simulink library "STATE_BIO_MASTER"  (Simulink 8.6)
settings: Solver=ode45  StartTime=0.0  StopTime=10.0  RelTol=1e-3
libraries: cdsBitwise x48, cdsEpicsIn x41, cdsFunctionCall x10, cdsEpicsOut x7
(part 1 of 2)
settings Model: Creator=controls  LastModifiedBy=controls

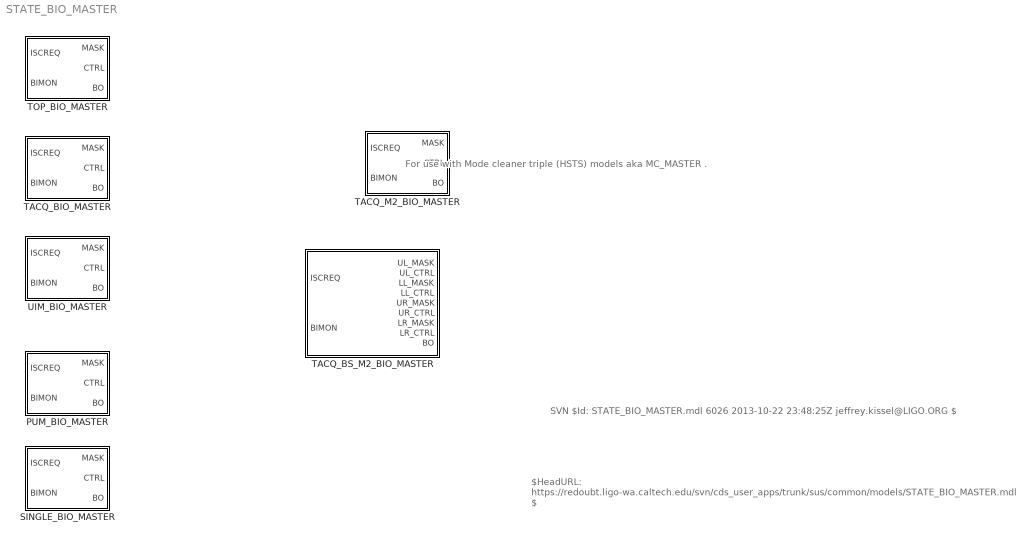
== system STATE_BIO_MASTER ==
  note: $HeadURL: https://redoubt.ligo-wa.caltech.edu/svn/cds_user_apps/trunk/sus/common/models/STATE_BIO_MASTER.mdl $
  note: For use with Mode cleaner triple (HSTS) models aka MC_MASTER
      |
      |
      |
      |
      |
      |
      |
      |
      |
      | .
  note: SVN $Id: STATE_BIO_MASTER.mdl 6026 2013-10-22 23:48:25Z jeffrey.kissel@LIGO.ORG $
  PUM_BIO_MASTER : Subsystem
  SINGLE_BIO_MASTER : Subsystem
  TACQ_BIO_MASTER : Subsystem
  TACQ_BS_M2_BIO_MASTER : Subsystem
  TACQ_M2_BIO_MASTER : Subsystem
  TOP_BIO_MASTER : Subsystem
  UIM_BIO_MASTER : Subsystem

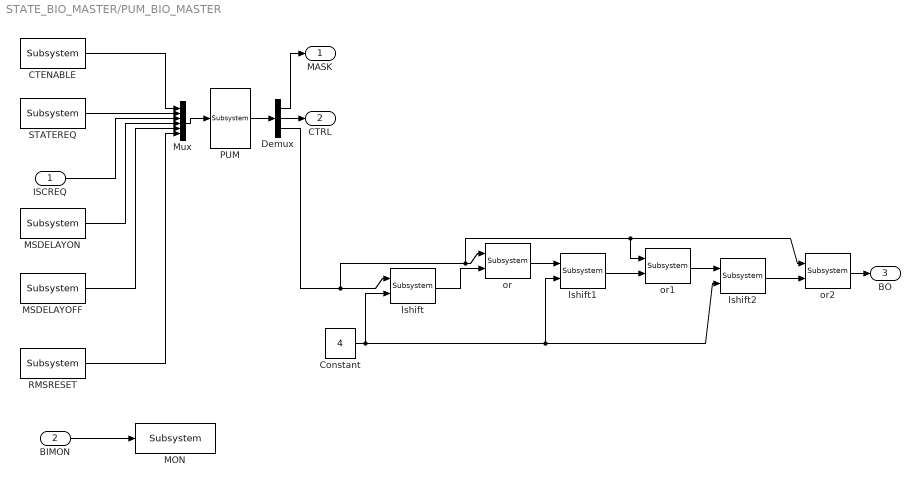
== system STATE_BIO_MASTER/PUM_BIO_MASTER ==
  ISCREQ : Inport
  BIMON : Inport  Port=2
  CTENABLE : cdsEpicsIn/Subsystem  Tag=cdsEpicsIn  Description=|
      | Purpose:                                                                              
      | Create an EPICS input channel connection to the FE realtime controls.                 
      |                                                                                       
      | Operation:                                                                            
      | Outputs value from an EPICS ai record. Value is floating point with a precision of 3..
      |                                                                                       
      | Usage:                                                                                
      | Name the part with the desired EPICS channel name.
      settings: AttributesFormatString=%<Tag>
  Constant : Constant  Value=4
  Demux : Demux  Outputs=3
  MON : cdsEpicsOut/Subsystem  Tag=cdsEpicsOutput  Description=|
      | Purpose:                                          
      | Output a FE signal to an EPICS channel.           
      |                                                   
      | Operation:                                        
      | Takes input value and passes it to EPICS record.  
      |                                                   
      | Usage:                                            
      | Name the part with the desired EPICS rrecord name.
      settings: AttributesFormatString=%<Tag>
  MSDELAYOFF : cdsEpicsIn/Subsystem  Tag=cdsEpicsIn  Description=|
      | Purpose:                                                                              
      | Create an EPICS input channel connection to the FE realtime controls.                 
      |                                                                                       
      | Operation:                                                                            
      | Outputs value from an EPICS ai record. Value is floating point with a precision of 3..
      |                                                                                       
      | Usage:                                                                                
      | Name the part with the desired EPICS channel name.
      settings: AttributesFormatString=%<Tag>
  MSDELAYON : cdsEpicsIn/Subsystem  Tag=cdsEpicsIn  Description=|
      | Purpose:                                                                              
      | Create an EPICS input channel connection to the FE realtime controls.                 
      |                                                                                       
      | Operation:                                                                            
      | Outputs value from an EPICS ai record. Value is floating point with a precision of 3..
      |                                                                                       
      | Usage:                                                                                
      | Name the part with the desired EPICS channel name.
      settings: AttributesFormatString=%<Tag>
  Mux : Mux  Inputs=6
  PUM : cdsFunctionCall/Subsystem  Tag=cdsFunctionCall  Description=inline PUM $SUS_SRC/CD_STATE_MACHINE.c
      settings: AttributesFormatString=%<Tag>
  RMSRESET : cdsEpicsIn/Subsystem  Tag=cdsEpicsIn  Description=|
      | Purpose:                                                                              
      | Create an EPICS input channel connection to the FE realtime controls.                 
      |                                                                                       
      | Operation:                                                                            
      | Outputs value from an EPICS ai record. Value is floating point with a precision of 3..
      |                                                                                       
      | Usage:                                                                                
      | Name the part with the desired EPICS channel name.
      settings: AttributesFormatString=%<Tag>
  STATEREQ : cdsEpicsIn/Subsystem  Tag=cdsEpicsIn  Description=|
      | Purpose:                                                                              
      | Create an EPICS input channel connection to the FE realtime controls.                 
      |                                                                                       
      | Operation:                                                                            
      | Outputs value from an EPICS ai record. Value is floating point with a precision of 3..
      |                                                                                       
      | Usage:                                                                                
      | Name the part with the desired EPICS channel name.
      settings: AttributesFormatString=%<Tag>
  lshift : cdsBitwise/Subsystem  Tag=cdsBitwise
      settings: AttributesFormatString=%<Tag>
  lshift1 : cdsBitwise/Subsystem  Tag=cdsBitwise
      settings: AttributesFormatString=%<Tag>
  lshift2 : cdsBitwise/Subsystem  Tag=cdsBitwise
      settings: AttributesFormatString=%<Tag>
  or : cdsBitwise/Subsystem  Tag=cdsBitwise
      settings: AttributesFormatString=%<Tag>
  or1 : cdsBitwise/Subsystem  Tag=cdsBitwise
      settings: AttributesFormatString=%<Tag>
  or2 : cdsBitwise/Subsystem  Tag=cdsBitwise
      settings: AttributesFormatString=%<Tag>
  MASK : Outport
  CTRL : Outport  Port=2
  BO : Outport  Port=3
  wires:
  PUM/1 -> Demux/1
  Mux/1 -> PUM/1
  CTENABLE/1 -> Mux/1
  STATEREQ/1 -> Mux/2
  ISCREQ/1 -> Mux/3
  MSDELAYON/1 -> Mux/4
  Demux/1 -> MASK/1
  Demux/2 -> CTRL/1
  BIMON/1 -> MON/1
  RMSRESET/1 -> Mux/6
  MSDELAYOFF/1 -> Mux/5
  Constant/1 -> lshift/2, lshift1/2, lshift2/2
  lshift/1 -> or/2
  or/1 -> lshift1/1
  lshift1/1 -> or1/2
  or1/1 -> lshift2/1
  lshift2/1 -> or2/2
  Demux/3 -> lshift/1, or/1, or1/1, or2/1
  or2/1 -> BO/1

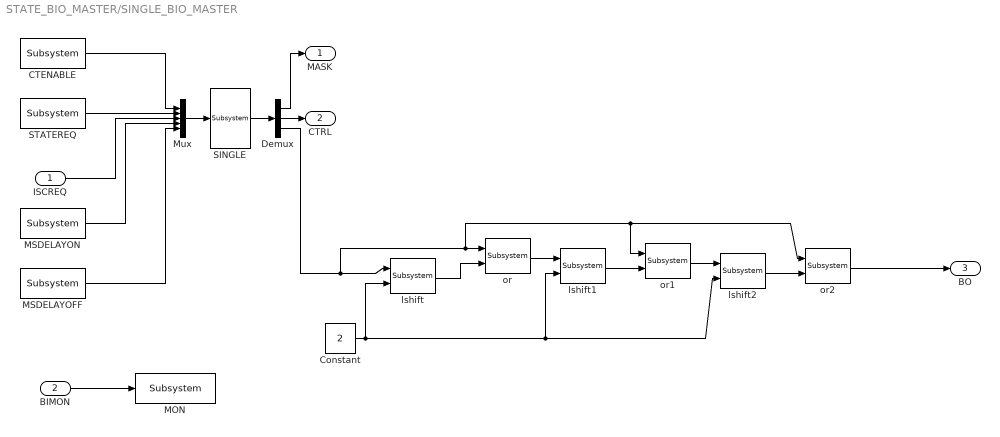
== system STATE_BIO_MASTER/SINGLE_BIO_MASTER ==
  ISCREQ : Inport
  BIMON : Inport  Port=2
  CTENABLE : cdsEpicsIn/Subsystem  Tag=cdsEpicsIn  Description=|
      | Purpose:                                                                              
      | Create an EPICS input channel connection to the FE realtime controls.                 
      |                                                                                       
      | Operation:                                                                            
      | Outputs value from an EPICS ai record. Value is floating point with a precision of 3..
      |                                                                                       
      | Usage:                                                                                
      | Name the part with the desired EPICS channel name.
      settings: AttributesFormatString=%<Tag>
  Constant : Constant  Value=2
  Demux : Demux  Outputs=3
  MON : cdsEpicsOut/Subsystem  Tag=cdsEpicsOutput  Description=|
      | Purpose:                                          
      | Output a FE signal to an EPICS channel.           
      |                                                   
      | Operation:                                        
      | Takes input value and passes it to EPICS record.  
      |                                                   
      | Usage:                                            
      | Name the part with the desired EPICS rrecord name.
      settings: AttributesFormatString=%<Tag>
  MSDELAYOFF : cdsEpicsIn/Subsystem  Tag=cdsEpicsIn  Description=|
      | Purpose:                                                                              
      | Create an EPICS input channel connection to the FE realtime controls.                 
      |                                                                                       
      | Operation:                                                                            
      | Outputs value from an EPICS ai record. Value is floating point with a precision of 3..
      |                                                                                       
      | Usage:                                                                                
      | Name the part with the desired EPICS channel name.
      settings: AttributesFormatString=%<Tag>
  MSDELAYON : cdsEpicsIn/Subsystem  Tag=cdsEpicsIn  Description=|
      | Purpose:                                                                              
      | Create an EPICS input channel connection to the FE realtime controls.                 
      |                                                                                       
      | Operation:                                                                            
      | Outputs value from an EPICS ai record. Value is floating point with a precision of 3..
      |                                                                                       
      | Usage:                                                                                
      | Name the part with the desired EPICS channel name.
      settings: AttributesFormatString=%<Tag>
  Mux : Mux  Inputs=5
  SINGLE : cdsFunctionCall/Subsystem  Tag=cdsFunctionCall  Description=inline SINGLE $SUS_SRC/CD_STATE_MACHINE.c
      settings: AttributesFormatString=%<Tag>
  STATEREQ : cdsEpicsIn/Subsystem  Tag=cdsEpicsIn  Description=|
      | Purpose:                                                                              
      | Create an EPICS input channel connection to the FE realtime controls.                 
      |                                                                                       
      | Operation:                                                                            
      | Outputs value from an EPICS ai record. Value is floating point with a precision of 3..
      |                                                                                       
      | Usage:                                                                                
      | Name the part with the desired EPICS channel name.
      settings: AttributesFormatString=%<Tag>
  lshift : cdsBitwise/Subsystem  Tag=cdsBitwise
      settings: AttributesFormatString=%<Tag>
  lshift1 : cdsBitwise/Subsystem  Tag=cdsBitwise
      settings: AttributesFormatString=%<Tag>
  lshift2 : cdsBitwise/Subsystem  Tag=cdsBitwise
      settings: AttributesFormatString=%<Tag>
  or : cdsBitwise/Subsystem  Tag=cdsBitwise
      settings: AttributesFormatString=%<Tag>
  or1 : cdsBitwise/Subsystem  Tag=cdsBitwise
      settings: AttributesFormatString=%<Tag>
  or2 : cdsBitwise/Subsystem  Tag=cdsBitwise
      settings: AttributesFormatString=%<Tag>
  MASK : Outport
  CTRL : Outport  Port=2
  BO : Outport  Port=3
  wires:
  Demux/3 -> or1/1, or2/1, or/1, lshift/1
  Demux/2 -> CTRL/1
  lshift2/1 -> or2/2
  or1/1 -> lshift2/1
  lshift1/1 -> or1/2
  or/1 -> lshift1/1
  lshift/1 -> or/2
  Constant/1 -> lshift/2, lshift1/2, lshift2/2
  MSDELAYOFF/1 -> Mux/5
  SINGLE/1 -> Demux/1
  Mux/1 -> SINGLE/1
  CTENABLE/1 -> Mux/1
  STATEREQ/1 -> Mux/2
  ISCREQ/1 -> Mux/3
  MSDELAYON/1 -> Mux/4
  Demux/1 -> MASK/1
  BIMON/1 -> MON/1
  or2/1 -> BO/1

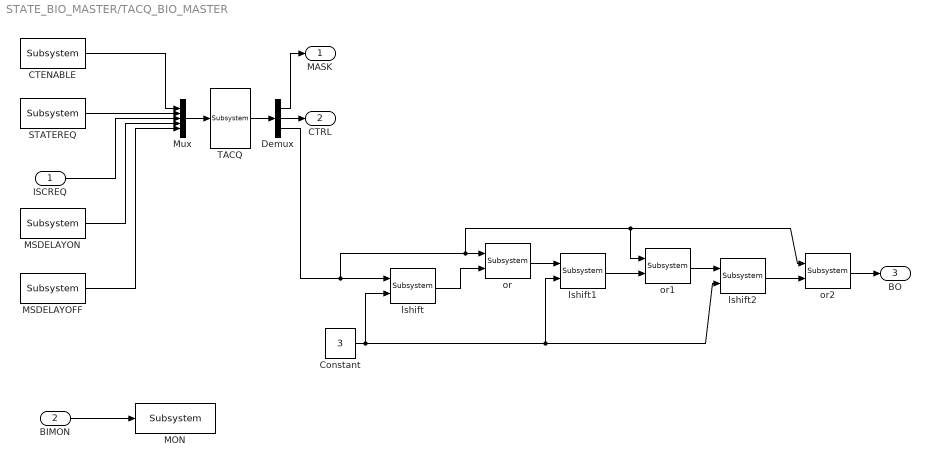
== system STATE_BIO_MASTER/TACQ_BIO_MASTER ==
  ISCREQ : Inport
  BIMON : Inport  Port=2
  CTENABLE : cdsEpicsIn/Subsystem  Tag=cdsEpicsIn  Description=|
      | Purpose:                                                                              
      | Create an EPICS input channel connection to the FE realtime controls.                 
      |                                                                                       
      | Operation:                                                                            
      | Outputs value from an EPICS ai record. Value is floating point with a precision of 3..
      |                                                                                       
      | Usage:                                                                                
      | Name the part with the desired EPICS channel name.
      settings: AttributesFormatString=%<Tag>
  Constant : Constant  Value=3
  Demux : Demux  Outputs=3
  MON : cdsEpicsOut/Subsystem  Tag=cdsEpicsOutput  Description=|
      | Purpose:                                          
      | Output a FE signal to an EPICS channel.           
      |                                                   
      | Operation:                                        
      | Takes input value and passes it to EPICS record.  
      |                                                   
      | Usage:                                            
      | Name the part with the desired EPICS rrecord name.
      settings: AttributesFormatString=%<Tag>
  MSDELAYOFF : cdsEpicsIn/Subsystem  Tag=cdsEpicsIn  Description=|
      | Purpose:                                                                              
      | Create an EPICS input channel connection to the FE realtime controls.                 
      |                                                                                       
      | Operation:                                                                            
      | Outputs value from an EPICS ai record. Value is floating point with a precision of 3..
      |                                                                                       
      | Usage:                                                                                
      | Name the part with the desired EPICS channel name.
      settings: AttributesFormatString=%<Tag>
  MSDELAYON : cdsEpicsIn/Subsystem  Tag=cdsEpicsIn  Description=|
      | Purpose:                                                                              
      | Create an EPICS input channel connection to the FE realtime controls.                 
      |                                                                                       
      | Operation:                                                                            
      | Outputs value from an EPICS ai record. Value is floating point with a precision of 3..
      |                                                                                       
      | Usage:                                                                                
      | Name the part with the desired EPICS channel name.
      settings: AttributesFormatString=%<Tag>
  Mux : Mux  Inputs=5
  STATEREQ : cdsEpicsIn/Subsystem  Tag=cdsEpicsIn  Description=|
      | Purpose:                                                                              
      | Create an EPICS input channel connection to the FE realtime controls.                 
      |                                                                                       
      | Operation:                                                                            
      | Outputs value from an EPICS ai record. Value is floating point with a precision of 3..
      |                                                                                       
      | Usage:                                                                                
      | Name the part with the desired EPICS channel name.
      settings: AttributesFormatString=%<Tag>
  TACQ : cdsFunctionCall/Subsystem  Tag=cdsFunctionCall  Description=inline TACQ /opt/rtcds/userapps/trunk/vis/common/src/CD_STATE_MACHINE.c
      settings: AttributesFormatString=%<Tag>
  lshift : cdsBitwise/Subsystem  Tag=cdsBitwise
      settings: AttributesFormatString=%<Tag>
  lshift1 : cdsBitwise/Subsystem  Tag=cdsBitwise
      settings: AttributesFormatString=%<Tag>
  lshift2 : cdsBitwise/Subsystem  Tag=cdsBitwise
      settings: AttributesFormatString=%<Tag>
  or : cdsBitwise/Subsystem  Tag=cdsBitwise
      settings: AttributesFormatString=%<Tag>
  or1 : cdsBitwise/Subsystem  Tag=cdsBitwise
      settings: AttributesFormatString=%<Tag>
  or2 : cdsBitwise/Subsystem  Tag=cdsBitwise
      settings: AttributesFormatString=%<Tag>
  MASK : Outport
  CTRL : Outport  Port=2
  BO : Outport  Port=3
  wires:
  TACQ/1 -> Demux/1
  Mux/1 -> TACQ/1
  CTENABLE/1 -> Mux/1
  STATEREQ/1 -> Mux/2
  ISCREQ/1 -> Mux/3
  MSDELAYON/1 -> Mux/4
  Demux/1 -> MASK/1
  Demux/2 -> CTRL/1
  BIMON/1 -> MON/1
  MSDELAYOFF/1 -> Mux/5
  Constant/1 -> lshift/2, lshift1/2, lshift2/2
  lshift/1 -> or/2
  or/1 -> lshift1/1
  lshift1/1 -> or1/2
  or1/1 -> lshift2/1
  lshift2/1 -> or2/2
  Demux/3 -> lshift/1, or/1, or1/1, or2/1
  or2/1 -> BO/1

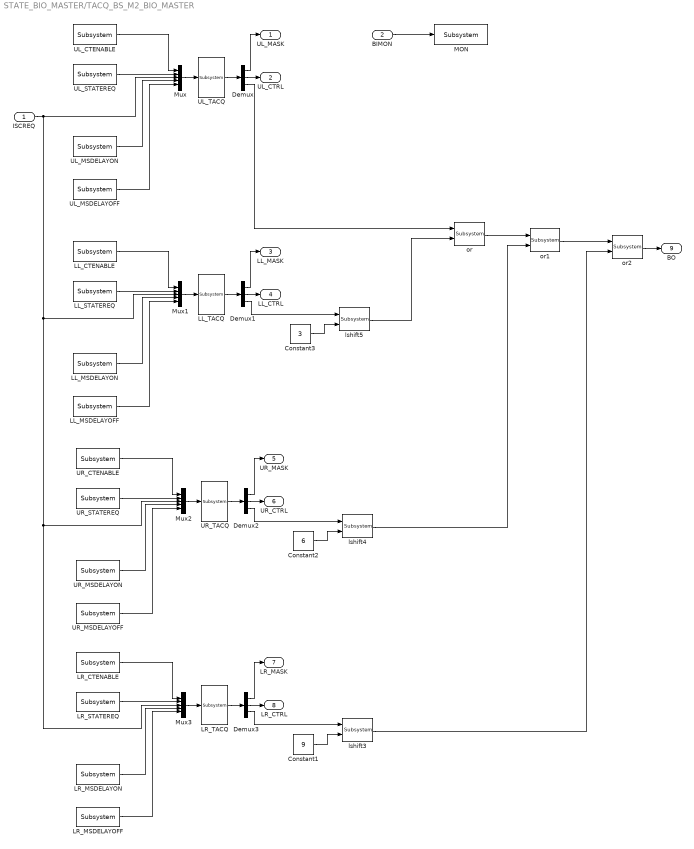
== system STATE_BIO_MASTER/TACQ_BS_M2_BIO_MASTER ==
  ISCREQ : Inport
  BIMON : Inport  Port=2
  Constant1 : Constant  Value=9
  Constant2 : Constant  Value=6
  Constant3 : Constant  Value=3
  Demux{,1..3} (4 alike) : Demux  Outputs=3
  LL_CTENABLE : cdsEpicsIn/Subsystem  Tag=cdsEpicsIn  Description=|
      | Purpose:                                                                              
      | Create an EPICS input channel connection to the FE realtime controls.                 
      |                                                                                       
      | Operation:                                                                            
      | Outputs value from an EPICS ai record. Value is floating point with a precision of 3..
      |                                                                                       
      | Usage:                                                                                
      | Name the part with the desired EPICS channel name.
      settings: AttributesFormatString=%<Tag>
  LL_MSDELAYOFF : cdsEpicsIn/Subsystem  Tag=cdsEpicsIn  Description=|
      | Purpose:                                                                              
      | Create an EPICS input channel connection to the FE realtime controls.                 
      |                                                                                       
      | Operation:                                                                            
      | Outputs value from an EPICS ai record. Value is floating point with a precision of 3..
      |                                                                                       
      | Usage:                                                                                
      | Name the part with the desired EPICS channel name.
      settings: AttributesFormatString=%<Tag>
  LL_MSDELAYON : cdsEpicsIn/Subsystem  Tag=cdsEpicsIn  Description=|
      | Purpose:                                                                              
      | Create an EPICS input channel connection to the FE realtime controls.                 
      |                                                                                       
      | Operation:                                                                            
      | Outputs value from an EPICS ai record. Value is floating point with a precision of 3..
      |                                                                                       
      | Usage:                                                                                
      | Name the part with the desired EPICS channel name.
      settings: AttributesFormatString=%<Tag>
  LL_STATEREQ : cdsEpicsIn/Subsystem  Tag=cdsEpicsIn  Description=|
      | Purpose:                                                                              
      | Create an EPICS input channel connection to the FE realtime controls.                 
      |                                                                                       
      | Operation:                                                                            
      | Outputs value from an EPICS ai record. Value is floating point with a precision of 3..
      |                                                                                       
      | Usage:                                                                                
      | Name the part with the desired EPICS channel name.
      settings: AttributesFormatString=%<Tag>
  LL_TACQ : cdsFunctionCall/Subsystem  Tag=cdsFunctionCall  Description=inline TACQ inline TACQ /opt/rtcds/userapps/trunk/vis/common/src/CD_STATE_MACHINE.c
      settings: AttributesFormatString=%<Tag>
  LR_CTENABLE : cdsEpicsIn/Subsystem  Tag=cdsEpicsIn  Description=|
      | Purpose:                                                                              
      | Create an EPICS input channel connection to the FE realtime controls.                 
      |                                                                                       
      | Operation:                                                                            
      | Outputs value from an EPICS ai record. Value is floating point with a precision of 3..
      |                                                                                       
      | Usage:                                                                                
      | Name the part with the desired EPICS channel name.
      settings: AttributesFormatString=%<Tag>
  LR_MSDELAYOFF : cdsEpicsIn/Subsystem  Tag=cdsEpicsIn  Description=|
      | Purpose:                                                                              
      | Create an EPICS input channel connection to the FE realtime controls.                 
      |                                                                                       
      | Operation:                                                                            
      | Outputs value from an EPICS ai record. Value is floating point with a precision of 3..
      |                                                                                       
      | Usage:                                                                                
      | Name the part with the desired EPICS channel name.
      settings: AttributesFormatString=%<Tag>
  LR_MSDELAYON : cdsEpicsIn/Subsystem  Tag=cdsEpicsIn  Description=|
      | Purpose:                                                                              
      | Create an EPICS input channel connection to the FE realtime controls.                 
      |                                                                                       
      | Operation:                                                                            
      | Outputs value from an EPICS ai record. Value is floating point with a precision of 3..
      |                                                                                       
      | Usage:                                                                                
      | Name the part with the desired EPICS channel name.
      settings: AttributesFormatString=%<Tag>
  LR_STATEREQ : cdsEpicsIn/Subsystem  Tag=cdsEpicsIn  Description=|
      | Purpose:                                                                              
      | Create an EPICS input channel connection to the FE realtime controls.                 
      |                                                                                       
      | Operation:                                                                            
      | Outputs value from an EPICS ai record. Value is floating point with a precision of 3..
      |                                                                                       
      | Usage:                                                                                
      | Name the part with the desired EPICS channel name.
      settings: AttributesFormatString=%<Tag>
  LR_TACQ : cdsFunctionCall/Subsystem  Tag=cdsFunctionCall  Description=inline TACQ $SUS_SRC/CD_STATE_MACHINE.c
      settings: AttributesFormatString=%<Tag>
  MON : cdsEpicsOut/Subsystem  Tag=cdsEpicsOutput  Description=|
      | Purpose:                                          
      | Output a FE signal to an EPICS channel.           
      |                                                   
      | Operation:                                        
      | Takes input value and passes it to EPICS record.  
      |                                                   
      | Usage:                                            
      | Name the part with the desired EPICS rrecord name.
      settings: AttributesFormatString=%<Tag>
  Mux{,1..3} (4 alike) : Mux  Inputs=5
  UL_CTENABLE : cdsEpicsIn/Subsystem  Tag=cdsEpicsIn  Description=|
      | Purpose:                                                                              
      | Create an EPICS input channel connection to the FE realtime controls.                 
      |                                                                                       
      | Operation:                                                                            
      | Outputs value from an EPICS ai record. Value is floating point with a precision of 3..
      |                                                                                       
      | Usage:                                                                                
      | Name the part with the desired EPICS channel name.
      settings: AttributesFormatString=%<Tag>
  UL_MSDELAYOFF : cdsEpicsIn/Subsystem  Tag=cdsEpicsIn  Description=|
      | Purpose:                                                                              
      | Create an EPICS input channel connection to the FE realtime controls.                 
      |                                                                                       
      | Operation:                                                                            
      | Outputs value from an EPICS ai record. Value is floating point with a precision of 3..
      |                                                                                       
      | Usage:                                                                                
      | Name the part with the desired EPICS channel name.
      settings: AttributesFormatString=%<Tag>
  UL_MSDELAYON : cdsEpicsIn/Subsystem  Tag=cdsEpicsIn  Description=|
      | Purpose:                                                                              
      | Create an EPICS input channel connection to the FE realtime controls.                 
      |                                                                                       
      | Operation:                                                                            
      | Outputs value from an EPICS ai record. Value is floating point with a precision of 3..
      |                                                                                       
      | Usage:                                                                                
      | Name the part with the desired EPICS channel name.
      settings: AttributesFormatString=%<Tag>
  UL_STATEREQ : cdsEpicsIn/Subsystem  Tag=cdsEpicsIn  Description=|
      | Purpose:                                                                              
      | Create an EPICS input channel connection to the FE realtime controls.                 
      |                                                                                       
      | Operation:                                                                            
      | Outputs value from an EPICS ai record. Value is floating point with a precision of 3..
      |                                                                                       
      | Usage:                                                                                
      | Name the part with the desired EPICS channel name.
      settings: AttributesFormatString=%<Tag>
  UL_TACQ : cdsFunctionCall/Subsystem  Tag=cdsFunctionCall  Description=inline TACQ inline TACQ /opt/rtcds/userapps/trunk/vis/common/src/CD_STATE_MACHINE.c
      settings: AttributesFormatString=%<Tag>
  UR_CTENABLE : cdsEpicsIn/Subsystem  Tag=cdsEpicsIn  Description=|
      | Purpose:                                                                              
      | Create an EPICS input channel connection to the FE realtime controls.                 
      |                                                                                       
      | Operation:                                                                            
      | Outputs value from an EPICS ai record. Value is floating point with a precision of 3..
      |                                                                                       
      | Usage:                                                                                
      | Name the part with the desired EPICS channel name.
      settings: AttributesFormatString=%<Tag>
  UR_MSDELAYOFF : cdsEpicsIn/Subsystem  Tag=cdsEpicsIn  Description=|
      | Purpose:                                                                              
      | Create an EPICS input channel connection to the FE realtime controls.                 
      |                                                                                       
      | Operation:                                                                            
      | Outputs value from an EPICS ai record. Value is floating point with a precision of 3..
      |                                                                                       
      | Usage:                                                                                
      | Name the part with the desired EPICS channel name.
      settings: AttributesFormatString=%<Tag>
  UR_MSDELAYON : cdsEpicsIn/Subsystem  Tag=cdsEpicsIn  Description=|
      | Purpose:                                                                              
      | Create an EPICS input channel connection to the FE realtime controls.                 
      |                                                                                       
      | Operation:                                                                            
      | Outputs value from an EPICS ai record. Value is floating point with a precision of 3..
      |                                                                                       
      | Usage:                                                                                
      | Name the part with the desired EPICS channel name.
      settings: AttributesFormatString=%<Tag>
  UR_STATEREQ : cdsEpicsIn/Subsystem  Tag=cdsEpicsIn  Description=|
      | Purpose:                                                                              
      | Create an EPICS input channel connection to the FE realtime controls.                 
      |                                                                                       
      | Operation:                                                                            
      | Outputs value from an EPICS ai record. Value is floating point with a precision of 3..
      |                                                                                       
      | Usage:                                                                                
      | Name the part with the desired EPICS channel name.
      settings: AttributesFormatString=%<Tag>
  UR_TACQ : cdsFunctionCall/Subsystem  Tag=cdsFunctionCall  Description=inline TACQ inline TACQ /opt/rtcds/userapps/trunk/vis/common/src/CD_STATE_MACHINE.c
      settings: AttributesFormatString=%<Tag>
  lshift3 : cdsBitwise/Subsystem  Tag=cdsBitwise
      settings: AttributesFormatString=%<Tag>
  lshift4 : cdsBitwise/Subsystem  Tag=cdsBitwise
      settings: AttributesFormatString=%<Tag>
  lshift5 : cdsBitwise/Subsystem  Tag=cdsBitwise
      settings: AttributesFormatString=%<Tag>
  or : cdsBitwise/Subsystem  Tag=cdsBitwise
      settings: AttributesFormatString=%<Tag>
  or1 : cdsBitwise/Subsystem  Tag=cdsBitwise
      settings: AttributesFormatString=%<Tag>
  or2 : cdsBitwise/Subsystem  Tag=cdsBitwise
      settings: AttributesFormatString=%<Tag>
  UL_MASK : Outport
  UL_CTRL : Outport  Port=2
  LL_MASK : Outport  Port=3
  LL_CTRL : Outport  Port=4
  UR_MASK : Outport  Port=5
  UR_CTRL : Outport  Port=6
  LR_MASK : Outport  Port=7
  LR_CTRL : Outport  Port=8
  BO : Outport  Port=9
  wires:
  or2/1 -> BO/1
  Demux/3 -> or/1
  UL_MSDELAYOFF/1 -> Mux/5
  BIMON/1 -> MON/1
  Demux/2 -> UL_CTRL/1
  Demux/1 -> UL_MASK/1
  UL_MSDELAYON/1 -> Mux/4
  ISCREQ/1 -> Mux3/3, Mux2/3, Mux1/3, Mux/3
  UL_STATEREQ/1 -> Mux/2
  UL_CTENABLE/1 -> Mux/1
  Mux/1 -> UL_TACQ/1
  UL_TACQ/1 -> Demux/1
  LL_MSDELAYOFF/1 -> Mux1/5
  Demux1/2 -> LL_CTRL/1
  Demux1/1 -> LL_MASK/1
  LL_MSDELAYON/1 -> Mux1/4
  LL_STATEREQ/1 -> Mux1/2
  LL_CTENABLE/1 -> Mux1/1
  Mux1/1 -> LL_TACQ/1
  LL_TACQ/1 -> Demux1/1
  UR_MSDELAYOFF/1 -> Mux2/5
  Demux2/2 -> UR_CTRL/1
  Demux2/1 -> UR_MASK/1
  UR_MSDELAYON/1 -> Mux2/4
  UR_STATEREQ/1 -> Mux2/2
  UR_CTENABLE/1 -> Mux2/1
  Mux2/1 -> UR_TACQ/1
  UR_TACQ/1 -> Demux2/1
  LR_MSDELAYOFF/1 -> Mux3/5
  Demux3/2 -> LR_CTRL/1
  Demux3/1 -> LR_MASK/1
  LR_MSDELAYON/1 -> Mux3/4
  LR_STATEREQ/1 -> Mux3/2
  LR_CTENABLE/1 -> Mux3/1
  Mux3/1 -> LR_TACQ/1
  LR_TACQ/1 -> Demux3/1
  Demux3/3 -> lshift3/1
  Constant1/1 -> lshift3/2
  Demux2/3 -> lshift4/1
  Constant2/1 -> lshift4/2
  Demux1/3 -> lshift5/1
  Constant3/1 -> lshift5/2
  lshift5/1 -> or/2
  lshift4/1 -> or1/2
  or/1 -> or1/1
  lshift3/1 -> or2/2
  or1/1 -> or2/1

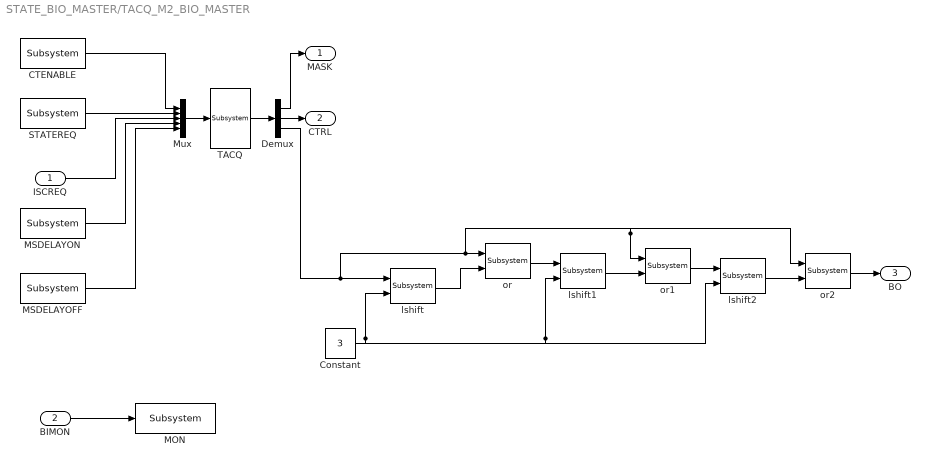
== system STATE_BIO_MASTER/TACQ_M2_BIO_MASTER ==
  ISCREQ : Inport
  BIMON : Inport  Port=2
  CTENABLE : cdsEpicsIn/Subsystem  Tag=cdsEpicsIn  Description=|  SystemSampleTime=-1
      | Purpose:                                                                              
      | Create an EPICS input channel connection to the FE realtime controls.                 
      |                                                                                       
      | Operation:                                                                            
      | Outputs value from an EPICS ai record. Value is floating point with a precision of 3..
      |                                                                                       
      | Usage:                                                                                
      | Name the part with the desired EPICS channel name.
      settings: AttributesFormatString=%<Tag>
  Constant : Constant  Value=3
  Demux : Demux  Outputs=3
  MON : cdsEpicsOut/Subsystem  Tag=cdsEpicsOutput  Description=|  SystemSampleTime=-1
      | Purpose:                                          
      | Output a FE signal to an EPICS channel.           
      |                                                   
      | Operation:                                        
      | Takes input value and passes it to EPICS record.  
      |                                                   
      | Usage:                                            
      | Name the part with the desired EPICS rrecord name.
      settings: AttributesFormatString=%<Tag>
  MSDELAYOFF : cdsEpicsIn/Subsystem  Tag=cdsEpicsIn  Description=|  SystemSampleTime=-1
      | Purpose:                                                                              
      | Create an EPICS input channel connection to the FE realtime controls.                 
      |                                                                                       
      | Operation:                                                                            
      | Outputs value from an EPICS ai record. Value is floating point with a precision of 3..
      |                                                                                       
      | Usage:                                                                                
      | Name the part with the desired EPICS channel name.
      settings: AttributesFormatString=%<Tag>
  MSDELAYON : cdsEpicsIn/Subsystem  Tag=cdsEpicsIn  Description=|  SystemSampleTime=-1
      | Purpose:                                                                              
      | Create an EPICS input channel connection to the FE realtime controls.                 
      |                                                                                       
      | Operation:                                                                            
      | Outputs value from an EPICS ai record. Value is floating point with a precision of 3..
      |                                                                                       
      | Usage:                                                                                
      | Name the part with the desired EPICS channel name.
      settings: AttributesFormatString=%<Tag>
  Mux : Mux  Inputs=5
  STATEREQ : cdsEpicsIn/Subsystem  Tag=cdsEpicsIn  Description=|  SystemSampleTime=-1
      | Purpose:                                                                              
      | Create an EPICS input channel connection to the FE realtime controls.                 
      |                                                                                       
      | Operation:                                                                            
      | Outputs value from an EPICS ai record. Value is floating point with a precision of 3..
      |                                                                                       
      | Usage:                                                                                
      | Name the part with the desired EPICS channel name.
      settings: AttributesFormatString=%<Tag>
  TACQ : cdsFunctionCall/Subsystem  Tag=cdsFunctionCall  Description=inline TACQ_M2 $SUS_SRC/CD_STATE_MACHINE.c  SystemSampleTime=-1
      settings: AttributesFormatString=%<Tag>
  lshift : cdsBitwise/Subsystem  Tag=cdsBitwise  SystemSampleTime=-1
      settings: AttributesFormatString=%<Tag>
  lshift1 : cdsBitwise/Subsystem  Tag=cdsBitwise  SystemSampleTime=-1
      settings: AttributesFormatString=%<Tag>
  lshift2 : cdsBitwise/Subsystem  Tag=cdsBitwise  SystemSampleTime=-1
      settings: AttributesFormatString=%<Tag>
  or : cdsBitwise/Subsystem  Tag=cdsBitwise  SystemSampleTime=-1
      settings: AttributesFormatString=%<Tag>
  or1 : cdsBitwise/Subsystem  Tag=cdsBitwise  SystemSampleTime=-1
      settings: AttributesFormatString=%<Tag>
  or2 : cdsBitwise/Subsystem  Tag=cdsBitwise  SystemSampleTime=-1
      settings: AttributesFormatString=%<Tag>
  MASK : Outport
  CTRL : Outport  Port=2
  BO : Outport  Port=3
  wires:
  or2/1 -> BO/1
  Demux/3 -> or2/1, or1/1, or/1, lshift/1
  lshift2/1 -> or2/2
  or1/1 -> lshift2/1
  lshift1/1 -> or1/2
  or/1 -> lshift1/1
  lshift/1 -> or/2
  Constant/1 -> lshift2/2, lshift1/2, lshift/2
  MSDELAYOFF/1 -> Mux/5
  BIMON/1 -> MON/1
  Demux/2 -> CTRL/1
  Demux/1 -> MASK/1
  MSDELAYON/1 -> Mux/4
  ISCREQ/1 -> Mux/3
  STATEREQ/1 -> Mux/2
  CTENABLE/1 -> Mux/1
  Mux/1 -> TACQ/1
  TACQ/1 -> Demux/1

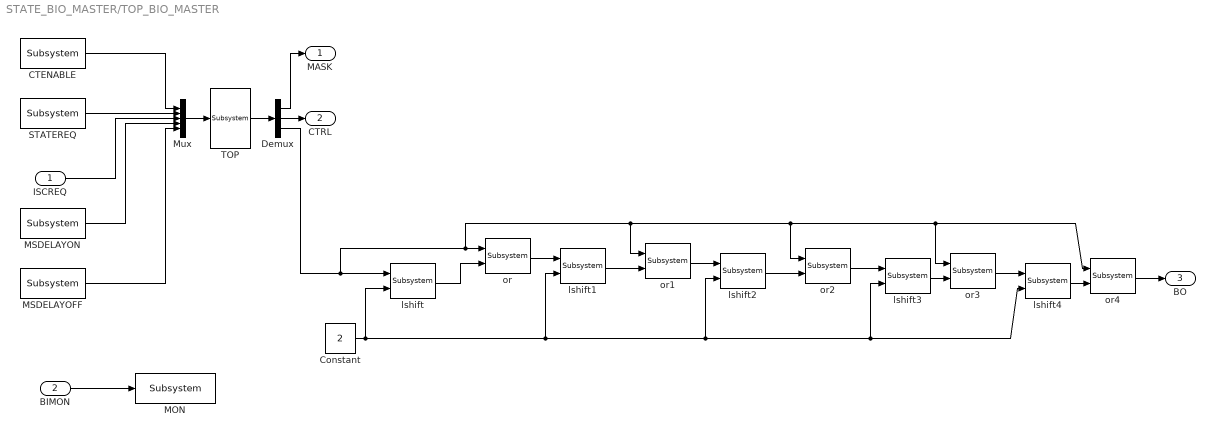
== system STATE_BIO_MASTER/TOP_BIO_MASTER ==
  ISCREQ : Inport
  BIMON : Inport  Port=2
  CTENABLE : cdsEpicsIn/Subsystem  Tag=cdsEpicsIn  Description=|
      | Purpose:                                                                              
      | Create an EPICS input channel connection to the FE realtime controls.                 
      |                                                                                       
      | Operation:                                                                            
      | Outputs value from an EPICS ai record. Value is floating point with a precision of 3..
      |                                                                                       
      | Usage:                                                                                
      | Name the part with the desired EPICS channel name.
      settings: AttributesFormatString=%<Tag>
  Constant : Constant  Value=2
  Demux : Demux  Outputs=3
  MON : cdsEpicsOut/Subsystem  Tag=cdsEpicsOutput  Description=|
      | Purpose:                                          
      | Output a FE signal to an EPICS channel.           
      |                                                   
      | Operation:                                        
      | Takes input value and passes it to EPICS record.  
      |                                                   
      | Usage:                                            
      | Name the part with the desired EPICS rrecord name.
      settings: AttributesFormatString=%<Tag>
  MSDELAYOFF : cdsEpicsIn/Subsystem  Tag=cdsEpicsIn  Description=|
      | Purpose:                                                                              
      | Create an EPICS input channel connection to the FE realtime controls.                 
      |                                                                                       
      | Operation:                                                                            
      | Outputs value from an EPICS ai record. Value is floating point with a precision of 3..
      |                                                                                       
      | Usage:                                                                                
      | Name the part with the desired EPICS channel name.
      settings: AttributesFormatString=%<Tag>
  MSDELAYON : cdsEpicsIn/Subsystem  Tag=cdsEpicsIn  Description=|
      | Purpose:                                                                              
      | Create an EPICS input channel connection to the FE realtime controls.                 
      |                                                                                       
      | Operation:                                                                            
      | Outputs value from an EPICS ai record. Value is floating point with a precision of 3..
      |                                                                                       
      | Usage:                                                                                
      | Name the part with the desired EPICS channel name.
      settings: AttributesFormatString=%<Tag>
  Mux : Mux  Inputs=5
  STATEREQ : cdsEpicsIn/Subsystem  Tag=cdsEpicsIn  Description=|
      | Purpose:                                                                              
      | Create an EPICS input channel connection to the FE realtime controls.                 
      |                                                                                       
      | Operation:                                                                            
      | Outputs value from an EPICS ai record. Value is floating point with a precision of 3..
      |                                                                                       
      | Usage:                                                                                
      | Name the part with the desired EPICS channel name.
      settings: AttributesFormatString=%<Tag>
  TOP : cdsFunctionCall/Subsystem  Tag=cdsFunctionCall  Description=inline TOP /opt/rtcds/userapps/trunk/vis/common/src/CD_STATE_MACHINE.c
      settings: AttributesFormatString=%<Tag>
  lshift{,1..4} (5 alike) : cdsBitwise/Subsystem  Tag=cdsBitwise
      settings: AttributesFormatString=%<Tag>
  or{,1..4} (5 alike) : cdsBitwise/Subsystem  Tag=cdsBitwise
      settings: AttributesFormatString=%<Tag>
  MASK : Outport
  CTRL : Outport  Port=2
  BO : Outport  Port=3
  wires:
  BIMON/1 -> MON/1
  Demux/1 -> MASK/1
  MSDELAYON/1 -> Mux/4
  ISCREQ/1 -> Mux/3
  STATEREQ/1 -> Mux/2
  CTENABLE/1 -> Mux/1
  Mux/1 -> TOP/1
  TOP/1 -> Demux/1
  MSDELAYOFF/1 -> Mux/5
  Constant/1 -> lshift/2, lshift1/2, lshift2/2, lshift3/2, lshift4/2
  lshift/1 -> or/2
  or/1 -> lshift1/1
  lshift1/1 -> or1/2
  or1/1 -> lshift2/1
  lshift2/1 -> or2/2
  or2/1 -> lshift3/1
  lshift3/1 -> or3/2
  or3/1 -> lshift4/1
  lshift4/1 -> or4/2
  Demux/2 -> CTRL/1
  or4/1 -> BO/1
  Demux/3 -> lshift/1, or/1, or1/1, or2/1, or3/1, or4/1
